simulink model "Attitude_Control_ADRC"  (R2016a)
settings: Solver=VariableStepAuto  StartTime=0.0  StopTime=20.0  FixedStep=0.005  RelTol=1e-3
settings Model: Creator=SRQ  LastModifiedBy=SRQ

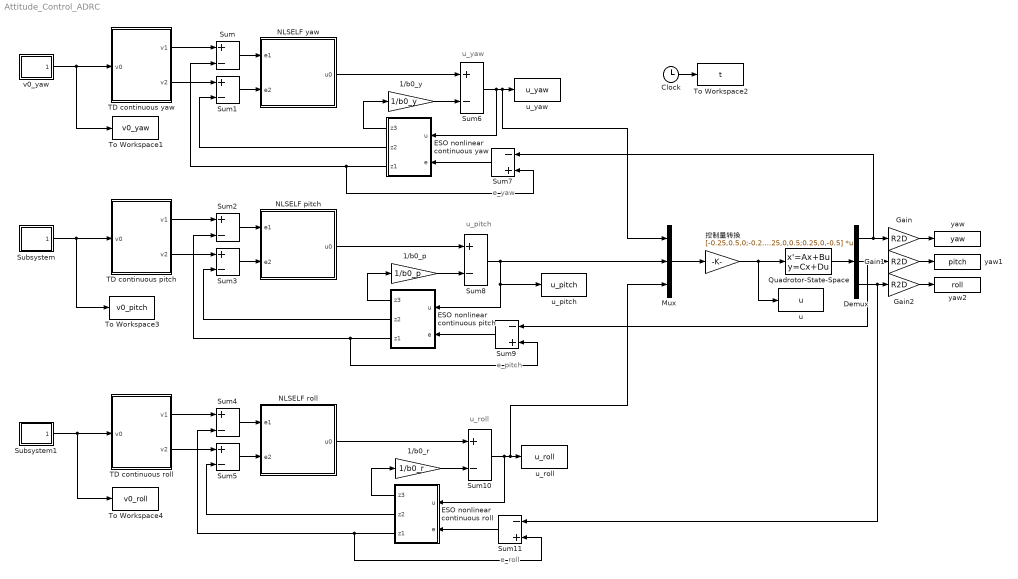
== system Attitude_Control_ADRC ==
  note: u_yaw
  note: u_pitch
  note: e_yaw
  note: e_pitch
  note: u_roll
  note: e_roll
  1/b0_p : Gain  Gain=1/b0_p  mask{b0_p=0.9}
  1/b0_r : Gain  Gain=1/b0_r  mask{b0_r=1.2}
  1/b0_y : Gain  Gain=1/b0_y  mask{b0_y=0.06}
  Clock : Clock
  Demux : Demux  Outputs=3
  ESO nonlinear continuous pitch : Subsystem
  ESO nonlinear continuous roll : Subsystem
  ESO nonlinear continuous yaw : Subsystem
  Gain : Gain  Gain=R2D  mask{R2D=180/pi}
  Gain1 : Gain  Gain=R2D  mask{R2D=180/pi}
  Gain2 : Gain  Gain=R2D  mask{R2D=180/pi}
  Mux : Mux  Inputs=3
  NLSELF pitch : Subsystem
  NLSELF roll : Subsystem
  NLSELF yaw : Subsystem
  Quadrotor-State-Space : StateSpace  A=[0,0,0,1,0,0;0,0,0,0,1,0;0,0,0,0,0,1;0,0,0,0,0,0;0,0,0,0,0,0;0,0,0,0,0,0]  B=[0,0,0,0;0,0,0,0;0,0,0,0;k_tc/J_y,k_tc/J_y,k_tn/J_y,k_tn/J_y;l*k_f/J_p,-l*k_f/J_p,0,0;0,0,l*k_f/J_r,-l*k_f/J_r]  C=[1,0,0,0,0,0;0,1,0,0,0,0;0,0,1,0,0,0]  D=[0,0,0,0;0,0,0,0;0,0,0,0]  X0=[-3*pi/180;-3*pi/180;-3*pi/180;0;0;0]  mask{k_tn=0.0036, k_tc=-0.0036, k_f=0.1188, J_y=0.1104, J_p=0.0552, J_r=0.0552, l=0.197}
      mask prompts: k_tn "k_tn 顺时针螺旋桨推力矩系数(N·m/V)"; k_tc "k_tc 逆时针螺旋桨推力矩系数(N·m/V)"; k_f "k_f 螺旋桨推力系数(N/V)"; J_y "J_y 偏航轴转动惯量(kg·m²)"; J_p "J_p 俯仰轴转动惯量(kg·m²)"; J_r "J_r 滚转轴转动惯量(kg·m²)"; l "l 旋转中心到螺旋桨中心的距离(m)"
  Subsystem : Subsystem
  Subsystem1 : Subsystem
  Sum{,1..6,8,10} (9 alike) : Sum  Inputs=+-
  Sum11 : Sum  Inputs=-+
  Sum7 : Sum  Inputs=-+
  Sum9 : Sum  Inputs=-+
  TD continuous pitch : Subsystem
  TD continuous roll : Subsystem
  TD continuous yaw : Subsystem
  To Workspace1 : ToWorkspace  VariableName=v0_yaw  SampleTime=-1
  To Workspace2 : ToWorkspace  VariableName=t  SampleTime=-1
  To Workspace3 : ToWorkspace  VariableName=v0_pitch  SampleTime=-1
  To Workspace4 : ToWorkspace  VariableName=v0_roll  SampleTime=-1
  u : ToWorkspace  VariableName=u  SampleTime=-1
  u_pitch : ToWorkspace  VariableName=u_pitch  SampleTime=-1
  u_roll : ToWorkspace  VariableName=u_roll  SampleTime=-1
  u_yaw : ToWorkspace  VariableName=u_yaw  SampleTime=-1
  v0_yaw : Subsystem
  yaw : ToWorkspace  VariableName=yaw  SampleTime=-1
  yaw1 : ToWorkspace  VariableName=pitch  SampleTime=-1
  yaw2 : ToWorkspace  VariableName=roll  SampleTime=-1
  控制量转换 : Gain  Gain=[-0.25,0.5,0;-0.25,-0.5,0;0.25,0,0.5;0.25,0,-0.5]  Multiplication=Matrix(K*u)
  wires:
  TD continuous yaw/1(v1) -> Sum/1
  TD continuous yaw/2(v2) -> Sum1/1
  Clock/1 -> To Workspace2/1
  TD continuous pitch/1(v1) -> Sum2/1
  TD continuous pitch/2(v2) -> Sum3/1
  TD continuous roll/1(v1) -> Sum4/1
  TD continuous roll/2(v2) -> Sum5/1
  Sum/1 -> NLSELF yaw/1(e1)
  Sum1/1 -> NLSELF yaw/2(e2)
  Sum2/1 -> NLSELF pitch/1(e1)
  Sum3/1 -> NLSELF pitch/2(e2)
  Sum4/1 -> NLSELF roll/1(e1)
  Sum5/1 -> NLSELF roll/2(e2)
  NLSELF yaw/1(u0) -> Sum6/1
  ESO nonlinear continuous yaw/3(z1) -> Sum7/2, Sum/2
  ESO nonlinear continuous yaw/2(z2) -> Sum1/2
  1/b0_y/1 -> Sum6/2
  ESO nonlinear continuous yaw/1(z3) -> 1/b0_y/1
  Sum6/1 -> ESO nonlinear continuous yaw/1(u), Mux/1, u_yaw/1
  Sum7/1 -> ESO nonlinear continuous yaw/2(e)
  NLSELF pitch/1(u0) -> Sum8/1
  ESO nonlinear continuous pitch/3(z1) -> Sum2/2, Sum9/2
  ESO nonlinear continuous pitch/2(z2) -> Sum3/2
  1/b0_p/1 -> Sum8/2
  ESO nonlinear continuous pitch/1(z3) -> 1/b0_p/1
  Sum8/1 -> Mux/2, ESO nonlinear continuous pitch/1(u), u_pitch/1
  Sum9/1 -> ESO nonlinear continuous pitch/2(e)
  NLSELF roll/1(u0) -> Sum10/1
  ESO nonlinear continuous roll/3(z1) -> Sum4/2, Sum11/2
  ESO nonlinear continuous roll/2(z2) -> Sum5/2
  1/b0_r/1 -> Sum10/2
  ESO nonlinear continuous roll/1(z3) -> 1/b0_r/1
  Sum10/1 -> ESO nonlinear continuous roll/1(u), Mux/3, u_roll/1
  Sum11/1 -> ESO nonlinear continuous roll/2(e)
  Mux/1 -> 控制量转换/1
  控制量转换/1 -> u/1, Quadrotor-State-Space/1
  Quadrotor-State-Space/1 -> Demux/1
  Demux/1 -> Sum7/1, Gain/1
  Demux/2 -> Sum9/1, Gain1/1
  Demux/3 -> Sum11/1, Gain2/1
  Gain/1 -> yaw/1
  Gain1/1 -> yaw1/1
  Gain2/1 -> yaw2/1
  v0_yaw/1(v0_yaw) -> To Workspace1/1, TD continuous yaw/1(v0)
  Subsystem/1(v0_pitch) -> To Workspace3/1, TD continuous pitch/1(v0)
  Subsystem1/1(v0_roll) -> To Workspace4/1, TD continuous roll/1(v0)

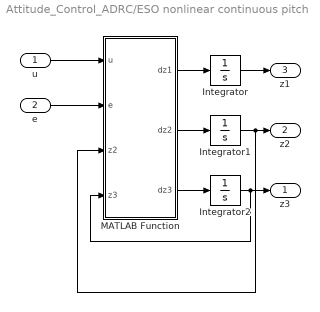
== system Attitude_Control_ADRC/ESO nonlinear continuous pitch ==
  u : Inport
  e : Inport  Port=2
  Integrator : Integrator
  Integrator1 : Integrator
  Integrator2 : Integrator
  MATLAB Function : MATLAB Function  TreatAsAtomicUnit=on
  z3 : Outport
  z2 : Outport  Port=2
  z1 : Outport  Port=3
  wires:
  Integrator/1 -> z1/1
  MATLAB Function/1(dz1) -> Integrator/1
  MATLAB Function/2(dz2) -> Integrator1/1
  Integrator1/1 -> MATLAB Function/3(z2), z2/1
  MATLAB Function/3(dz3) -> Integrator2/1
  Integrator2/1 -> MATLAB Function/4(z3), z3/1
  u/1 -> MATLAB Function/1(u)
  e/1 -> MATLAB Function/2(e)

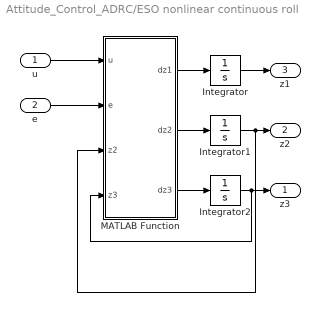
== system Attitude_Control_ADRC/ESO nonlinear continuous roll ==
  u : Inport
  e : Inport  Port=2
  Integrator : Integrator
  Integrator1 : Integrator
  Integrator2 : Integrator
  MATLAB Function : MATLAB Function  TreatAsAtomicUnit=on
  z3 : Outport
  z2 : Outport  Port=2
  z1 : Outport  Port=3
  wires:
  Integrator/1 -> z1/1
  MATLAB Function/1(dz1) -> Integrator/1
  MATLAB Function/2(dz2) -> Integrator1/1
  Integrator1/1 -> MATLAB Function/3(z2), z2/1
  MATLAB Function/3(dz3) -> Integrator2/1
  u/1 -> MATLAB Function/1(u)
  e/1 -> MATLAB Function/2(e)
  Integrator2/1 -> MATLAB Function/4(z3), z3/1

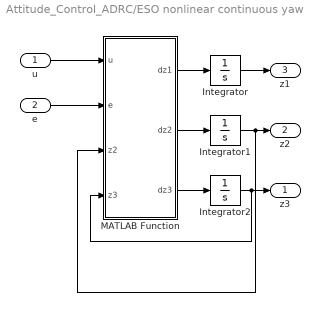
== system Attitude_Control_ADRC/ESO nonlinear continuous yaw ==
  u : Inport
  e : Inport  Port=2
  Integrator : Integrator
  Integrator1 : Integrator
  Integrator2 : Integrator
  MATLAB Function : MATLAB Function  TreatAsAtomicUnit=on
  z3 : Outport
  z2 : Outport  Port=2
  z1 : Outport  Port=3
  wires:
  Integrator/1 -> z1/1
  MATLAB Function/1(dz1) -> Integrator/1
  MATLAB Function/2(dz2) -> Integrator1/1
  Integrator1/1 -> MATLAB Function/3(z2), z2/1
  MATLAB Function/3(dz3) -> Integrator2/1
  u/1 -> MATLAB Function/1(u)
  e/1 -> MATLAB Function/2(e)
  Integrator2/1 -> MATLAB Function/4(z3), z3/1

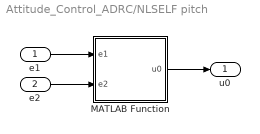
== system Attitude_Control_ADRC/NLSELF pitch ==
  e1 : Inport
  e2 : Inport  Port=2
  MATLAB Function : MATLAB Function  TreatAsAtomicUnit=on
  u0 : Outport
  wires:
  MATLAB Function/1(u0) -> u0/1
  e1/1 -> MATLAB Function/1(e1)
  e2/1 -> MATLAB Function/2(e2)

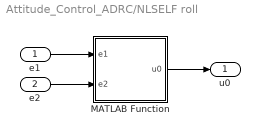
== system Attitude_Control_ADRC/NLSELF roll ==
  e1 : Inport
  e2 : Inport  Port=2
  MATLAB Function : MATLAB Function  TreatAsAtomicUnit=on
  u0 : Outport
  wires:
  MATLAB Function/1(u0) -> u0/1
  e1/1 -> MATLAB Function/1(e1)
  e2/1 -> MATLAB Function/2(e2)

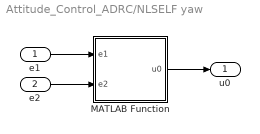
== system Attitude_Control_ADRC/NLSELF yaw ==
  e1 : Inport
  e2 : Inport  Port=2
  MATLAB Function : MATLAB Function  TreatAsAtomicUnit=on
  u0 : Outport
  wires:
  MATLAB Function/1(u0) -> u0/1
  e1/1 -> MATLAB Function/1(e1)
  e2/1 -> MATLAB Function/2(e2)

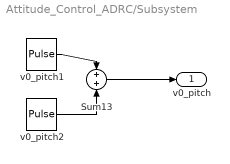
== system Attitude_Control_ADRC/Subsystem ==
  Sum13 : Sum
  v0_pitch1 : DiscretePulseGenerator  PulseType=Time based  Amplitude=3*pi/180  Period=10  PulseWidth=50  PhaseDelay=5
  v0_pitch2 : DiscretePulseGenerator  PulseType=Time based  Amplitude=-3*pi/180  Period=10  PulseWidth=50
  v0_pitch : Outport
  wires:
  v0_pitch1/1 -> Sum13/1
  v0_pitch2/1 -> Sum13/2
  Sum13/1 -> v0_pitch/1

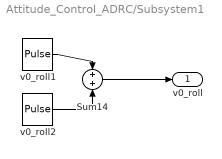
== system Attitude_Control_ADRC/Subsystem1 ==
  Sum14 : Sum
  v0_roll1 : DiscretePulseGenerator  PulseType=Time based  Amplitude=3*pi/180  Period=10  PulseWidth=50  PhaseDelay=5
  v0_roll2 : DiscretePulseGenerator  PulseType=Time based  Amplitude=-3*pi/180  Period=10  PulseWidth=50
  v0_roll : Outport
  wires:
  v0_roll2/1 -> Sum14/2
  v0_roll1/1 -> Sum14/1
  Sum14/1 -> v0_roll/1

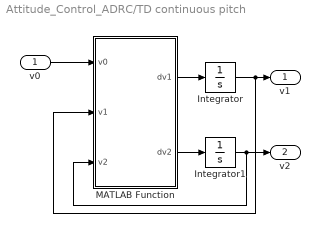
== system Attitude_Control_ADRC/TD continuous pitch ==
  v0 : Inport
  Integrator : Integrator
  Integrator1 : Integrator
  MATLAB Function : MATLAB Function  TreatAsAtomicUnit=on
  v1 : Outport
  v2 : Outport  Port=2
  wires:
  v0/1 -> MATLAB Function/1(v0)
  MATLAB Function/1(dv1) -> Integrator/1
  Integrator/1 -> MATLAB Function/2(v1), v1/1
  Integrator1/1 -> MATLAB Function/3(v2), v2/1
  MATLAB Function/2(dv2) -> Integrator1/1

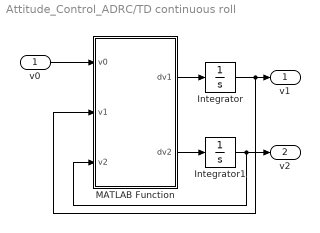
== system Attitude_Control_ADRC/TD continuous roll ==
  v0 : Inport
  Integrator : Integrator
  Integrator1 : Integrator
  MATLAB Function : MATLAB Function  TreatAsAtomicUnit=on
  v1 : Outport
  v2 : Outport  Port=2
  wires:
  v0/1 -> MATLAB Function/1(v0)
  MATLAB Function/1(dv1) -> Integrator/1
  Integrator/1 -> MATLAB Function/2(v1), v1/1
  Integrator1/1 -> MATLAB Function/3(v2), v2/1
  MATLAB Function/2(dv2) -> Integrator1/1

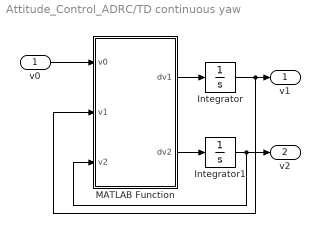
== system Attitude_Control_ADRC/TD continuous yaw ==
  v0 : Inport
  Integrator : Integrator
  Integrator1 : Integrator
  MATLAB Function : MATLAB Function  TreatAsAtomicUnit=on
  v1 : Outport
  v2 : Outport  Port=2
  wires:
  v0/1 -> MATLAB Function/1(v0)
  MATLAB Function/1(dv1) -> Integrator/1
  Integrator/1 -> MATLAB Function/2(v1), v1/1
  Integrator1/1 -> MATLAB Function/3(v2), v2/1
  MATLAB Function/2(dv2) -> Integrator1/1

== system Attitude_Control_ADRC/v0_yaw ==
  Sum12 : Sum
  v0_yaw1 : DiscretePulseGenerator  PulseType=Time based  Amplitude=3*pi/180  Period=10  PulseWidth=50  PhaseDelay=5
  v0_yaw2 : DiscretePulseGenerator  PulseType=Time based  Amplitude=-3*pi/180  Period=10  PulseWidth=50
  v0_yaw : Outport
  wires:
  v0_yaw2/1 -> Sum12/2
  Sum12/1 -> v0_yaw/1
  v0_yaw1/1 -> Sum12/1

== matlab function Attitude_Control_ADRC/TD continuous pitch/MATLAB Function ==
  data: v0 input; dv1 output; dv2 output; v1 input; v2 input
function [dv1, dv2] = fcn(v0, v1, v2)
%连续型跟踪微分器TD
%% 参数赋值
h0 = 0.05;            % 滤波因子
omega_p = 5;         % 决定跟踪快慢的参数
%% 连续形式的跟踪微分器算法
dv1 = v2;
dv2 = fst(v1-v0, v2, omega_p, h0);

== matlab function Attitude_Control_ADRC/TD continuous yaw/MATLAB Function ==
  data: v0 input; dv1 output; dv2 output; v1 input; v2 input
function [dv1, dv2] = fcn(v0, v1, v2)
%连续型跟踪微分器TD
%% 参数赋值
h0 = 0.05;            % 滤波因子
omega_y = 2;         % 决定跟踪快慢的参数
%% 连续形式的跟踪微分器算法
dv1 = v2;
dv2 = fst(v1-v0, v2, omega_y, h0);

== matlab function Attitude_Control_ADRC/TD continuous roll/MATLAB Function ==
  data: v0 input; dv1 output; dv2 output; v1 input; v2 input
function [dv1, dv2] = fcn(v0, v1, v2)
%连续型跟踪微分器TD
%% 参数赋值
h0 = 0.05;            % 滤波因子
omega_r = 5;         % 决定跟踪快慢的参数
%% 连续形式的跟踪微分器算法
dv1 = v2;
dv2 = fst(v1-v0, v2, omega_r, h0);

== matlab function Attitude_Control_ADRC/NLSELF yaw/MATLAB Function ==
  data: e1 input; u0 output; e2 input
function u0 = fcn(e1,e2)
%#非线性状态误差反馈律(NLSEF)

%% 参数赋值
beta1_y = 200;   % 可调参数
beta2_y = 120;   % 可调参数
delta_y = 1;     % 线性段的区间长度
a1 = 0.5;        % 可调参数
a2 = 0.05;       % 可调参数
%% 一种采用fal()函数组合的NLSEF算法
u0 = beta1_y * fal(e1, a1, delta_y) + beta2_y * fal(e2, a2, delta_y);

== matlab function Attitude_Control_ADRC/NLSELF pitch/MATLAB Function ==
  data: e1 input; u0 output; e2 input
function u0 = fcn(e1,e2)
%#非线性状态误差反馈律(NLSEF)

%% 参数赋值
beta1_p = 150;   % 可调参数
beta2_p = 120;   % 可调参数
delta_p = 3;     % 线性段的区间长度
a1 = 0.5;        % 可调参数
a2 = 0.05;       % 可调参数
%% 一种采用fal()函数组合的NLSEF算法
u0 = beta1_p * fal(e1, a1, delta_p) + beta2_p * fal(e2, a2, delta_p);

== matlab function Attitude_Control_ADRC/NLSELF roll/MATLAB Function ==
  data: e1 input; u0 output; e2 input
function u0 = fcn(e1,e2)
%#非线性状态误差反馈律(NLSEF)

%% 参数赋值
beta1_r = 180;   % 可调参数
beta2_r = 120;   % 可调参数
delta_r = 3;     % 线性段的区间长度
a1 = 0.5;        % 可调参数
a2 = 0.05;       % 可调参数
%% 一种采用fal()函数组合的NLSEF算法
u0 = beta1_r * fal(e1, a1, delta_r) + beta2_r * fal(e2, a2, delta_r);

== matlab function Attitude_Control_ADRC/ESO nonlinear continuous yaw/MATLAB Function ==
  data: dz1 output; dz2 output; dz3 output; u input; e input; z2 input; z3 input
function [dz1,dz2,dz3] = fcn(u,e,z2, z3)
%#连续形式的扩张状态观测器(ESO)

%% 参数赋值
beta01_y = 30;     % 可调参数
beta02_y = 300;     % 可调参数
beta03_y = 1000;   % 可调参数
a1 = 0.75;         % 可调参数
a2 = 0.5;          % 可调参数
a3 = 0.25;         % 可调参数
delta = 0.006;     % 线性段的区间长度
b0_y = 0.06;       % 决定补偿强弱的“补偿因子”

dz1 = z2 - beta01_y * fal(e, a1, delta);
dz2 = z3 - beta02_y * fal(e, a2, delta) + b0_y * u;
dz3 = - beta03_y * fal(e, a3, delta);

== matlab function Attitude_Control_ADRC/ESO nonlinear continuous pitch/MATLAB Function ==
  data: u input; dz1 output; e input; dz2 output; dz3 output; z2 input; z3 input
function [dz1,dz2,dz3] = fcn(u,e,z2, z3)
%#连续形式的扩张状态观测器(ESO)

%% 参数赋值
beta01_p = 30;     % 可调参数
beta02_p = 300;     % 可调参数
beta03_p = 1000;   % 可调参数
a1 = 0.75;         % 可调参数
a2 = 0.5;          % 可调参数
a3 = 0.25;         % 可调参数
delta = 0.006;     % 线性段的区间长度
b0_p = 0.9;       % 决定补偿强弱的“补偿因子”

dz1 = z2 - beta01_p * fal(e, a1, delta);
dz2 = z3 - beta02_p * fal(e, a2, delta) + b0_p * u;
dz3 = - beta03_p * fal(e, a3, delta);

== matlab function Attitude_Control_ADRC/ESO nonlinear continuous roll/MATLAB Function ==
  data: u input; dz1 output; e input; dz2 output; dz3 output; z2 input; z3 input
function [dz1,dz2,dz3] = fcn(u,e,z2, z3)
%#连续形式的扩张状态观测器(ESO)

%% 参数赋值
beta01_r = 30;     % 可调参数
beta02_r = 300;     % 可调参数
beta03_r = 1000;   % 可调参数
a1 = 0.75;         % 可调参数
a2 = 0.5;          % 可调参数
a3 = 0.25;         % 可调参数
delta = 0.006;     % 线性段的区间长度
b0_r = 1.2;       % 决定补偿强弱的“补偿因子”

dz1 = z2 - beta01_r * fal(e, a1, delta);
dz2 = z3 - beta02_r * fal(e, a2, delta) + b0_r * u;
dz3 = - beta03_r * fal(e, a3, delta);
